simulink model "cutting_Machine"  (R2019a)
settings: Solver=VariableStepAuto  StartTime=0.0  StopTime=1009  RelTol=1e-3
values from neighbouring files (symbols this model uses):
  B = 0.029    [cuttingMachine.m]
  J = 0.1    [cuttingMachine.m]
  Ke = 0.66    [cuttingMachine.m]
  Km = 0.66    [cuttingMachine.m]
  Kt = 0.66    [cuttingMachine.m]
  La = 0.001    [cuttingMachine.m]
  Ra = 1    [cuttingMachine.m]
settings Model: Creator=colas  LastModifiedBy=colas

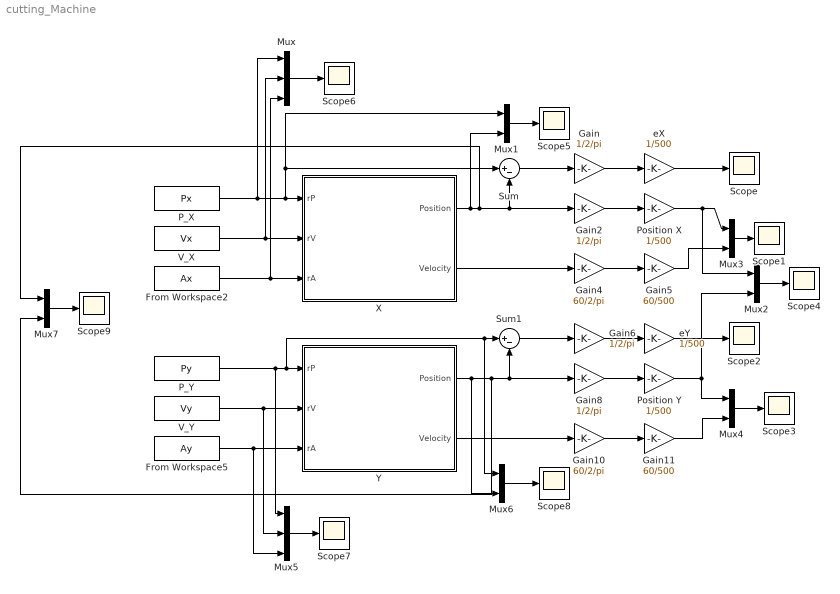
== system cutting_Machine ==
  From Workspace2 : FromWorkspace  VariableName=Ax  SampleTime=0
  From Workspace5 : FromWorkspace  VariableName=Ay  SampleTime=0
  Gain{,2,6,8} (4 alike) : Gain  Gain=1/2/pi
  Gain10 : Gain  Gain=60/2/pi
  Gain11 : Gain  Gain=60/500
  Gain4 : Gain  Gain=60/2/pi
  Gain5 : Gain  Gain=60/500
  Mux : Mux  Inputs=3
  Mux{1..4,6..7} (6 alike) : Mux  Inputs=2
  Mux5 : Mux  Inputs=3
  P_X : FromWorkspace  VariableName=Px  SampleTime=0
  P_Y : FromWorkspace  VariableName=Py  SampleTime=0
  Position X : Gain  Gain=1/500
  Position Y : Gain  Gain=1/500
  Scope{,1..9} (10 alike) : Scope
  Sum : Sum  Inputs=|+-
  Sum1 : Sum  Inputs=|+-
  V_X : FromWorkspace  VariableName=Vx  SampleTime=0
  V_Y : FromWorkspace  VariableName=Vy  SampleTime=0
  X : Subsystem
  Y : Subsystem
  eX : Gain  Gain=1/500
  eY : Gain  Gain=1/500
  wires:
  Sum/1 -> Gain/1
  Gain/1 -> eX/1
  Gain2/1 -> Position X/1
  X/2(Velocity) -> Gain4/1
  Gain4/1 -> Gain5/1
  eX/1 -> Scope/1
  Position X/1 -> Mux2/1, Mux3/1
  Gain11/1 -> Mux4/2
  Position Y/1 -> Mux2/2, Mux4/1
  eY/1 -> Scope2/1
  Gain10/1 -> Gain11/1
  Y/2(Velocity) -> Gain10/1
  Gain8/1 -> Position Y/1
  Gain6/1 -> eY/1
  Sum1/1 -> Gain6/1
  P_X/1 -> Mux/1, Mux1/1, Sum/1, X/1(rP)
  V_X/1 -> Mux/2, X/2(rV)
  From Workspace2/1 -> Mux/3, X/3(rA)
  Mux/1 -> Scope6/1
  Mux1/1 -> Scope5/1
  Mux2/1 -> Scope4/1
  Mux3/1 -> Scope1/1
  Gain5/1 -> Mux3/2
  Mux4/1 -> Scope3/1
  P_Y/1 -> Mux5/1, Mux6/1, Sum1/1, Y/1(rP)
  V_Y/1 -> Mux5/2, Y/2(rV)
  From Workspace5/1 -> Mux5/3, Y/3(rA)
  Mux5/1 -> Scope7/1
  Mux6/1 -> Scope8/1
  Mux7/1 -> Scope9/1
  Y/1(Position) -> Mux6/2, Mux7/2, Sum1/2, Gain8/1
  X/1(Position) -> Mux1/2, Mux7/1, Gain2/1, Sum/2

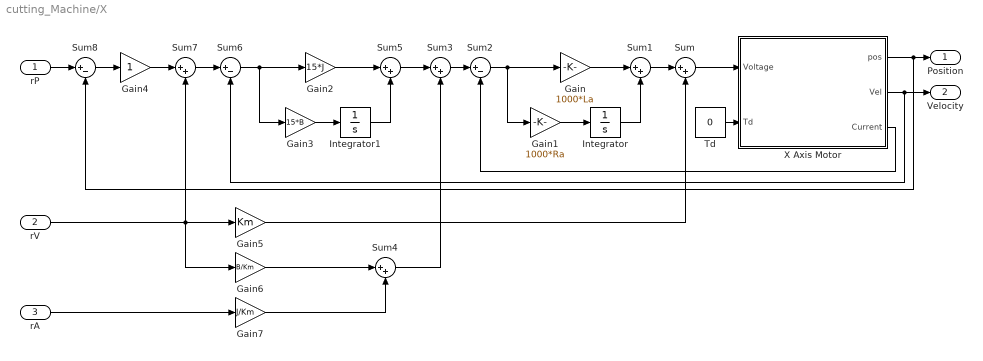
== system cutting_Machine/X ==
  rP : Inport
  rV : Inport  Port=2
  rA : Inport  Port=3
  Gain : Gain  Gain=1000*La
  Gain1 : Gain  Gain=1000*Ra
  Gain2 : Gain  Gain=15*J
  Gain3 : Gain  Gain=15*B
  Gain4 : Gain
  Gain5 : Gain  Gain=Km
  Gain6 : Gain  Gain=B/Km
  Gain7 : Gain  Gain=J/Km
  Integrator : Integrator
  Integrator1 : Integrator
  Sum{,1,3..5,7} (6 alike) : Sum  Inputs=|++
  Sum2 : Sum  Inputs=|+-
  Sum6 : Sum  Inputs=|+-
  Sum8 : Sum  Inputs=|+-
  Td : Constant  Value=0
  X Axis Motor : Subsystem
  Position : Outport
  Velocity : Outport  Port=2
  wires:
  X Axis Motor/3(Current) -> Sum2/2
  Sum2/1 -> Gain1/1, Gain/1
  Sum6/1 -> Gain3/1, Gain2/1
  rV/1 -> Gain6/1, Gain5/1, Sum7/2
  Gain6/1 -> Sum4/1
  Gain7/1 -> Sum4/2
  Sum4/1 -> Sum3/2
  rA/1 -> Gain7/1
  Sum/1 -> X Axis Motor/1(Voltage)
  Integrator/1 -> Sum1/2
  Sum1/1 -> Sum/1
  X Axis Motor/1(pos) -> Position/1, Sum8/2
  Gain5/1 -> Sum/2
  Gain/1 -> Sum1/1
  Sum8/1 -> Gain4/1
  Gain2/1 -> Sum5/1
  Sum5/1 -> Sum3/1
  Gain1/1 -> Integrator/1
  Integrator1/1 -> Sum5/2
  Sum3/1 -> Sum2/1
  rP/1 -> Sum8/1
  X Axis Motor/2(Vel) -> Velocity/1, Sum6/2
  Td/1 -> X Axis Motor/2(Td)
  Gain4/1 -> Sum7/1
  Sum7/1 -> Sum6/1
  Gain3/1 -> Integrator1/1

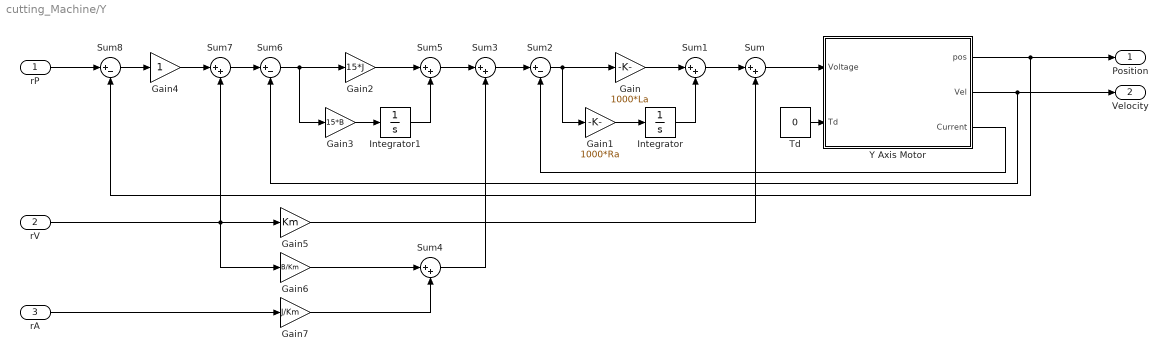
== system cutting_Machine/Y ==
  rP : Inport
  rV : Inport  Port=2
  rA : Inport  Port=3
  Gain : Gain  Gain=1000*La
  Gain1 : Gain  Gain=1000*Ra
  Gain2 : Gain  Gain=15*J
  Gain3 : Gain  Gain=15*B
  Gain4 : Gain
  Gain5 : Gain  Gain=Km
  Gain6 : Gain  Gain=B/Km
  Gain7 : Gain  Gain=J/Km
  Integrator : Integrator
  Integrator1 : Integrator
  Sum{,1,3..5,7} (6 alike) : Sum  Inputs=|++
  Sum2 : Sum  Inputs=|+-
  Sum6 : Sum  Inputs=|+-
  Sum8 : Sum  Inputs=|+-
  Td : Constant  Value=0
  Y Axis Motor : Subsystem
  Position : Outport
  Velocity : Outport  Port=2
  wires:
  Gain3/1 -> Integrator1/1
  Sum7/1 -> Sum6/1
  Gain4/1 -> Sum7/1
  Td/1 -> Y Axis Motor/2(Td)
  Y Axis Motor/2(Vel) -> Sum6/2, Velocity/1
  rP/1 -> Sum8/1
  Sum3/1 -> Sum2/1
  Integrator1/1 -> Sum5/2
  Gain1/1 -> Integrator/1
  Sum5/1 -> Sum3/1
  Gain2/1 -> Sum5/1
  Sum8/1 -> Gain4/1
  Gain/1 -> Sum1/1
  Gain5/1 -> Sum/2
  Y Axis Motor/1(pos) -> Sum8/2, Position/1
  Sum1/1 -> Sum/1
  Integrator/1 -> Sum1/2
  Sum/1 -> Y Axis Motor/1(Voltage)
  rA/1 -> Gain7/1
  Sum4/1 -> Sum3/2
  Gain7/1 -> Sum4/2
  Gain6/1 -> Sum4/1
  rV/1 -> Sum7/2, Gain5/1, Gain6/1
  Sum6/1 -> Gain2/1, Gain3/1
  Sum2/1 -> Gain/1, Gain1/1
  Y Axis Motor/3(Current) -> Sum2/2

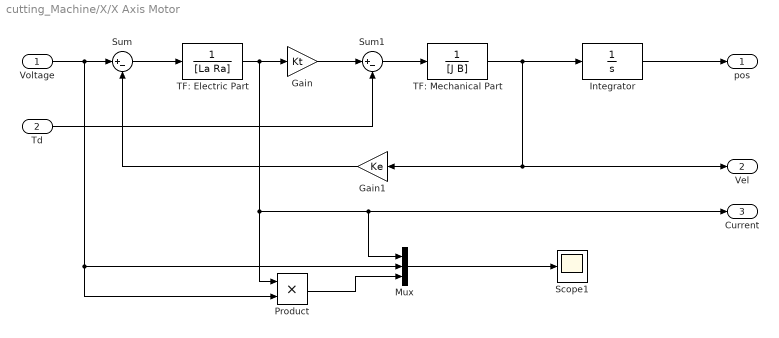
== system cutting_Machine/X/X Axis Motor ==
  Voltage : Inport
  Td : Inport  Port=2
  Gain : Gain  Gain=Kt
  Gain1 : Gain  Gain=Ke
  Integrator : TransferFcn  Denominator=[1 0]
  Mux : Mux  Inputs=3
  Product : Product
  Scope1 : Scope
  Sum : Sum  Inputs=|+-
  Sum1 : Sum  Inputs=|+-
  TF: Electric Part : TransferFcn  Denominator=[La Ra]
  TF: Mechanical Part : TransferFcn  Denominator=[J B]
  pos : Outport
  Vel : Outport  Port=2
  Current : Outport  Port=3
  wires:
  Gain1/1 -> Sum/2
  Integrator/1 -> pos/1
  Sum/1 -> TF: Electric Part/1
  TF: Mechanical Part/1 -> Vel/1, Gain1/1, Integrator/1
  Sum1/1 -> TF: Mechanical Part/1
  Voltage/1 -> Mux/2, Product/2, Sum/1
  Gain/1 -> Sum1/1
  Td/1 -> Sum1/2
  Mux/1 -> Scope1/1
  Product/1 -> Mux/3
  TF: Electric Part/1 -> Product/1, Mux/1, Current/1, Gain/1

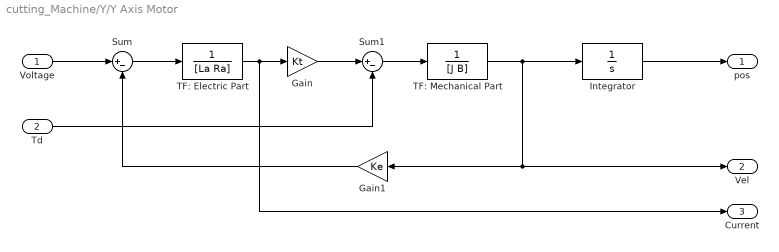
== system cutting_Machine/Y/Y Axis Motor ==
  Voltage : Inport
  Td : Inport  Port=2
  Gain : Gain  Gain=Kt
  Gain1 : Gain  Gain=Ke
  Integrator : TransferFcn  Denominator=[1 0]
  Sum : Sum  Inputs=|+-
  Sum1 : Sum  Inputs=|+-
  TF: Electric Part : TransferFcn  Denominator=[La Ra]
  TF: Mechanical Part : TransferFcn  Denominator=[J B]
  pos : Outport
  Vel : Outport  Port=2
  Current : Outport  Port=3
  wires:
  Td/1 -> Sum1/2
  Gain/1 -> Sum1/1
  Voltage/1 -> Sum/1
  Sum1/1 -> TF: Mechanical Part/1
  TF: Electric Part/1 -> Gain/1, Current/1
  TF: Mechanical Part/1 -> Integrator/1, Gain1/1, Vel/1
  Sum/1 -> TF: Electric Part/1
  Integrator/1 -> pos/1
  Gain1/1 -> Sum/2
